simulink model "drone_nonlinear_full_characterlistics"  (R2018a)
settings: Solver=VariableStepAuto  StartTime=0.0  StopTime=20  RelTol=1e-3
undefined symbols (not defined in the file): est_c_A, est_c_B, est_c_C, est_c_D, g, Ix, Iy, Iz, m
settings Model: Creator=ros  LastModifiedBy=ros

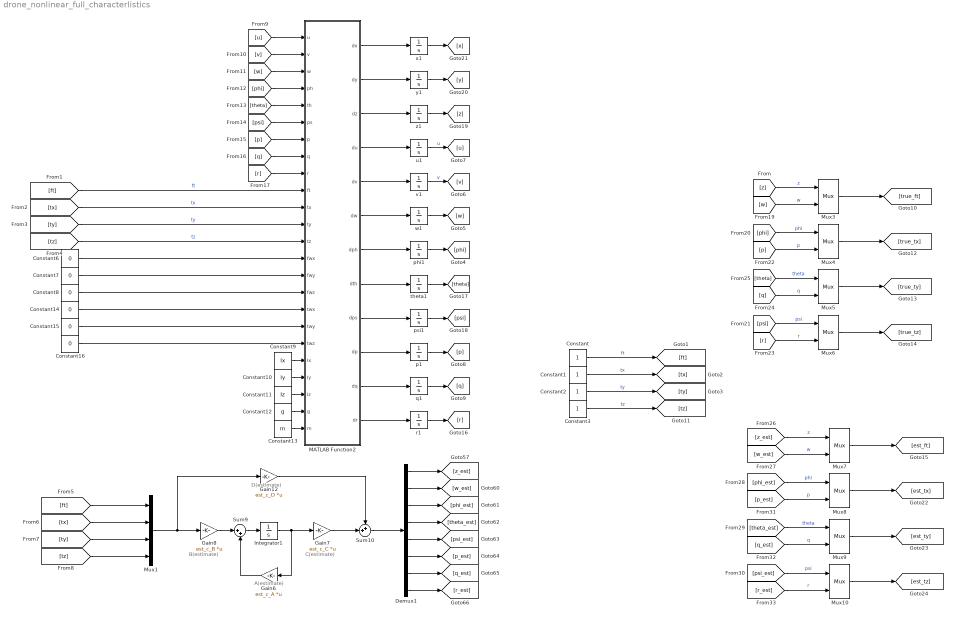
== system drone_nonlinear_full_characterlistics ==
  note: B(estimate)
  note: C(estimate)
  note: A(estimate)
  note: D(estimate)
  Constant{,1..3} (4 alike) : Constant
  Constant10 : Constant  Value=Iy
  Constant11 : Constant  Value=Iz
  Constant12 : Constant  Value=g
  Constant13 : Constant  Value=m
  Constant{6..8,14..16} (6 alike) : Constant  Value=0
  Constant9 : Constant  Value=Ix
  Demux1 : Demux  Outputs=8
  Gain12 : Gain  Gain=est_c_D  Multiplication=Matrix(K*u)
  Gain6 : Gain  Gain=est_c_A  Multiplication=Matrix(K*u)
  Gain7 : Gain  Gain=est_c_C  Multiplication=Matrix(K*u)
  Gain8 : Gain  Gain=est_c_B  Multiplication=Matrix(K*u)
  Integrator1 : Integrator
  MATLAB Function2 : MATLAB Function  TreatAsAtomicUnit=on
  Mux1 : Mux
  Mux{3..10} (8 alike) : Mux  Inputs=2
      settings: DisplayOption=signals
  Sum10 : Sum  Inputs=++|
  Sum9 : Sum  Inputs=|++
  p1 : Integrator
  phi1 : Integrator
  psi1 : Integrator
  q1 : Integrator
  r1 : Integrator
  theta1 : Integrator
  u1 : Integrator
  v1 : Integrator
  w1 : Integrator
  x1 : Integrator
  y1 : Integrator
  z1 : Integrator
  wires:
  [v] -> MATLAB Function2/2(v)
  MATLAB Function2/9(dps) -> psi1/1
  MATLAB Function2/10(dp) -> p1/1
  MATLAB Function2/5(dv) -> v1/1
  [r] -> MATLAB Function2/9(r)
  [psi] -> MATLAB Function2/6(ps)
  [p] -> MATLAB Function2/7(p)
  p1/1 -> [p]
  MATLAB Function2/12(dr) -> r1/1
  theta1/1 -> [theta]
  [w] -> MATLAB Function2/3(w)
  [phi] -> MATLAB Function2/4(ph)
  [q] -> MATLAB Function2/8(q)
  r1/1 -> [r]
  q1/1 -> [q]
  MATLAB Function2/11(dq) -> q1/1
  MATLAB Function2/6(dw) -> w1/1
  MATLAB Function2/4(du) -> u1/1
  psi1/1 -> [psi]
  [u] -> MATLAB Function2/1(u)
  MATLAB Function2/8(dth) -> theta1/1
  [theta] -> MATLAB Function2/5(th)
  u1/1 -> [u]  "u"
  w1/1 -> [w]
  MATLAB Function2/7(dph) -> phi1/1
  v1/1 -> [v]  "v"
  Constant9/1 -> MATLAB Function2/20(Ix)
  Constant13/1 -> MATLAB Function2/24(m)
  Constant11/1 -> MATLAB Function2/22(Iz)
  Constant10/1 -> MATLAB Function2/21(Iy)
  Constant12/1 -> MATLAB Function2/23(g)
  MATLAB Function2/1(dx) -> x1/1
  MATLAB Function2/2(dy) -> y1/1
  MATLAB Function2/3(dz) -> z1/1
  Constant6/1 -> MATLAB Function2/14(fwx)
  Constant7/1 -> MATLAB Function2/15(fwy)
  Constant14/1 -> MATLAB Function2/17(twx)
  Constant8/1 -> MATLAB Function2/16(fwz)
  Constant15/1 -> MATLAB Function2/18(twy)
  Constant16/1 -> MATLAB Function2/19(twz)
  z1/1 -> [z]
  y1/1 -> [y]
  x1/1 -> [x]
  phi1/1 -> [phi]
  [ft] -> MATLAB Function2/10(ft)  "ft"
  [tx] -> MATLAB Function2/11(tx)  "tx"
  [ty] -> MATLAB Function2/12(ty)  "ty"
  [tz] -> MATLAB Function2/13(tz)  "tz"
  Mux1/1 -> Gain12/1, Gain8/1
  Sum9/1 -> Integrator1/1
  Integrator1/1 -> Gain7/1, Gain6/1
  Gain8/1 -> Sum9/1
  Gain6/1 -> Sum9/2
  Gain7/1 -> Sum10/2
  Gain12/1 -> Sum10/1
  Sum10/1 -> Demux1/1
  Demux1/1 -> [z_est]
  Demux1/2 -> [w_est]
  Demux1/3 -> [phi_est]
  Demux1/4 -> [theta_est]
  Demux1/5 -> [psi_est]
  Demux1/6 -> [p_est]
  Demux1/7 -> [q_est]
  Demux1/8 -> [r_est]
  [ft] -> Mux1/1
  [tx] -> Mux1/2
  [ty] -> Mux1/3
  [tz] -> Mux1/4
  [z] -> Mux3/1  "z"
  [w] -> Mux3/2  "w"
  [phi] -> Mux4/1  "phi"
  [p] -> Mux4/2  "p"
  [theta] -> Mux5/1  "theta"
  [q] -> Mux5/2  "q"
  [psi] -> Mux6/1  "psi"
  [r] -> Mux6/2  "r"
  [w_est] -> Mux7/2  "w"
  [theta_est] -> Mux9/1  "theta"
  [z_est] -> Mux7/1  "z"
  [q_est] -> Mux9/2  "q"
  [phi_est] -> Mux8/1  "phi"
  [p_est] -> Mux8/2  "p"
  [r_est] -> Mux10/2  "r"
  [psi_est] -> Mux10/1  "psi"
  Mux3/1 -> [true_ft]
  Mux4/1 -> [true_tx]
  Mux5/1 -> [true_ty]
  Mux6/1 -> [true_tz]
  Mux10/1 -> [est_tz]
  Mux9/1 -> [est_ty]
  Mux8/1 -> [est_tx]
  Mux7/1 -> [est_ft]
  Constant/1 -> [ft]  "ft"
  Constant1/1 -> [tx]  "tx"
  Constant2/1 -> [ty]  "ty"
  Constant3/1 -> [tz]  "tz"

== matlab function drone_nonlinear_full_characterlistics/MATLAB Function2 ==
  data: u input; v input; dx output; w input; ph input; th input; ps input; p input; q input; r input; ft input; tx input; ty input; tz input; fwx input; fwy input; fwz input; twx input; twy input; twz input; dy output; dz output; du output; dv output; dw output; dph output; dth output; dps output; dp output; dq output; dr output; Ix input; Iy input; Iz input; g input; m input
function [dx, dy, dz, du, dv, dw, dph, dth, dps, dp, dq, dr] = fcn(u, v, w, ph, th, ps, p, q, r, ft, tx, ty, tz, fwx, fwy, fwz, twx, twy, twz, Ix, Iy, Iz, g, m)

dx = w*(sin(ph)*sin(ps) + cos(ph)*cos(ps)*sin(th)) - v*(cos(ph)*sin(ps) - cos(ps)*sin(ph)*sin(th)) + u*(cos(ps)*cos(th));
dy = v*(cos(ph)*cos(ps) + sin(ph)*sin(ps)*sin(th)) - w*(cos(ps)*sin(ph) - cos(ph)*sin(ps)*sin(th)) + u*(cos(th)*sin(ps));
dz = w*(cos(ph)*cos(th)) - u*(sin(th)) + v*(cos(th)*sin(ph));
du = r*v - q*w + g*(sin(th)) + fwx / m;
dv = p*w - r*u - g*(sin(ph)*cos(th)) + fwy / m;
dw = q*u - p*v - g*(cos(th)*cos(ph)) + (fwz + ft) / m;
dph = p + r*(cos(ph)*tan(th)) + q*(sin(ph)*tan(th));
dth = q*(cos(th)) - r*(sin(ph));
dps = r*(cos(ph)/cos(th)) + q*(sin(ph)/cos(th));
dp = r*q*(Iy - Iz)/Ix + (tx + twx)/Ix;
dq = p*r*(Iz - Ix)/Iy + (ty + twy)/Iy;
dr = p*q*(Ix - Iy)/Iz + (tz + twz)/Iz;
